simulink model "example_husky"  (R2024b)
settings: Solver=VariableStepAuto  StartTime=0.0  StopTime=inf  RelTol=1e-3
undefined symbols (not defined in the file): gray
settings Model: Creator=tsamak  LastModifiedBy=tsamak
settings OptimizationCC: ZeroExternalMemoryAtStartup=off  ZeroInternalMemoryAtStartup=off  InitFltsAndDblsToZero=on
settings DebuggingCC: UnderSpecifiedDimensionMsg=warning
settings HardwareCC: ProdLongLongMode=on  TargetLongLongMode=on
settings SFSimCC: SimTargetLang=C++  GPUAcceleration=on  SimDLTargetLibrary=cudnn
settings RTWCC: TargetLang=C++  GenerateGPUCode=CUDA  GPUComputeCapability=3.5
settings GRTTargetCC: TargetLangStandard=C++11 (ISO)  CodeInterfacePackaging=C++ class

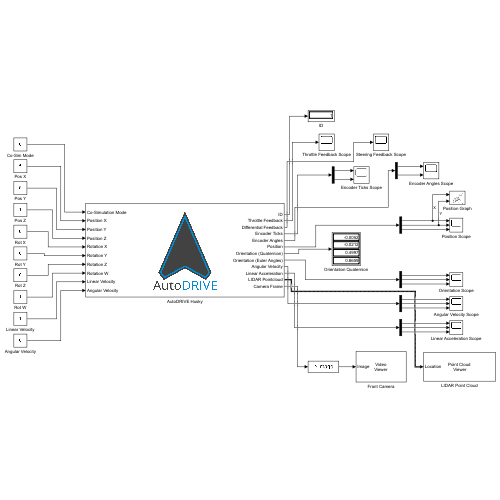
[thumbnail: Simulink's stored preview of the top-level diagram]
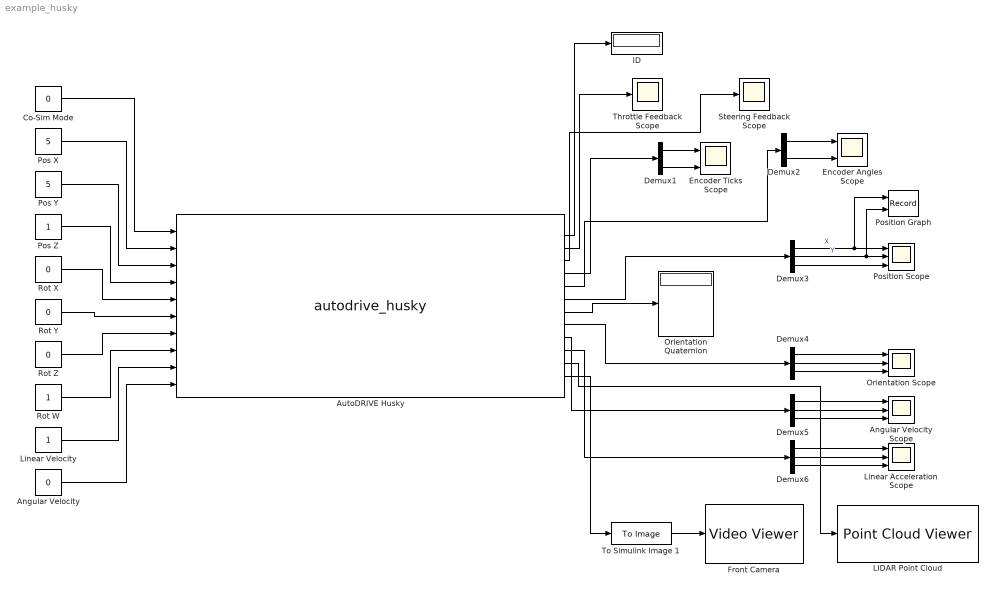
== system example_husky ==
  Angular Velocity : Constant  Value=0
  Angular Velocity Scope : Scope  NumInputPorts=3
  AutoDRIVE Husky : M-S-Function  FunctionName=autodrive_husky  Parameters=Port  mask{Port=4567}
      mask Display:
      | image('autodrive_logo.png');
      | port_label('input', 1, 'Co-Simulation Mode');
      | port_label('input', 2, 'Position X');
      | port_label('input', 3, 'Position Y');
      | port_label('input', 4, 'Position Z');
      | port_label('input', 5, 'Rotation X');
      | port_label('input', 6, 'Rotation Y');
      | port_label('input', 7, 'Rotation Z');
      | port_label('input', 8, 'Rotation W');
      | port_label('input', 9, 'Linear Velocity');
      | port_label('input', 10, 'Angular Velocity');
      | port_label('output', 1, 'ID');
      | port_label('output', 2, 'Throttle Feedback');
      | port_label('output', 3, 'Differential Feedback');
      | port_label('output', 4, 'Encoder Ticks');
      | port_label('output', 5, 'Encoder Angles');
      | port_label('output', 6, 'Position');
      | port_label('output', 7, 'Orientation (Quaternion)');
      | port_label('output', 8, 'Orientation (Euler Angles)');
      | port_label('output', 9, 'Angular Velocity');
      | port_label('output', 10, 'Linear Acceleration');
      | port_label('output', 11, 'LIDAR Pointcloud');
      | port_label('output', 12, 'Camera Frame');
  Co-Sim Mode : Constant  Value=0  OutDataTypeStr=uint8
  Demux1 : Demux  Outputs=2
  Demux2 : Demux  Outputs=2
  Demux{3..6} (4 alike) : Demux  Outputs=3
  Encoder Angles Scope : Scope  NumInputPorts=2
  Encoder Ticks Scope : Scope  NumInputPorts=2
  Front Camera : VideoViewer  colormapValue=gray(256)  FigPos=[11 410 408 304]
  ID : Display
  LIDAR Point Cloud : PointCloudViewer  FigPos=[843.666666666667 412 469.333333333333 328.666666666667]
  Linear Acceleration Scope : Scope  NumInputPorts=3
  Linear Velocity : Constant
  Orientation Quaternion : Display
  Orientation Scope : Scope  NumInputPorts=3
  Pos X : Constant  Value=5
  Pos Y : Constant  Value=5
  Pos Z : Constant
  Position Graph : Record  FileSettingsInternal="{\"entries\":[{\"content\":{\"excelSettings\":{\"content\":{},\"type\":\"Streamout.ExcelSettings\"}},\"type\":\"Streamout.FileSettingStorage\",\"uuid\":\"\"}],\"packageUris\":[\"http:\\/\\/schema.mathworks.com\\/mf0\\/streamout_blocks\\/R2020a\"],\"version\":\"1.0\"}"  Layout=[1 1]  SignalsInternal="{\"entries\":[{\"content\":{\"signals\":[{\"content\":{\"blockPath\":[],\"dimensions\":[1,1],\"domain\":\"\",\"lineColor\":\"#139fff\",\"plots\":[ 1 ],\"port\":1,\"sid\":[\"\"],\"signalID\":1,\"signalName\":\"X\"},\"type\":\"RecordBlkView.Signal\",\"uuid\":\"\"},{\"content\":{\"blockPath\":[],\"dimensions\":[1,1],\"domain\":\"\",\"lineColor\":\"#139fff\",\"plots\":[ 1 ],\"port\":2,\"sid\":[\"\"],\"signalID\":2,\"signalName\":\"Y\"},\"type\":\"RecordBlkView.Signal\",\"uuid\":\"\"}]},\"type\":\"RecordBlkView.InputSignals\",\"uuid\":\"\"}],\"packageUris\":[\"http:\\/\\/schema.mathworks.com\\/mf0\\/streamout_blocks\\/R2020a\"],\"version\":\"1.0\"}"  VisualizationBindings="{\"xyplotplugin\":{\"info\":[{\"series\":[{\"bindingParametersList\":[{\"parameter\":\"X-Axis\",\"signalID\":1,\"signalName\":\"X\"},{\"parameter\":\"Y-Axis\",\"signalID\":2,\"signalName\":\"Y\"}],\"seriesID\":0}],\"subplotID\":1}]}}"  CompatibilityTag=XY
  Position Scope : Scope  NumInputPorts=3
  Rot W : Constant
  Rot X : Constant  Value=0
  Rot Y : Constant  Value=0
  Rot Z : Constant  Value=0
  Steering Feedback Scope : Scope
  Throttle Feedback Scope : Scope
  To Simulink Image 1 : ToImage
  wires:
  Linear Velocity/1 -> AutoDRIVE Husky/9
  Angular Velocity/1 -> AutoDRIVE Husky/10
  Demux3/2 -> Position Scope/2, Position Graph/2  "Y"
  Demux3/1 -> Position Scope/1, Position Graph/1  "X"
  Demux3/3 -> Position Scope/3
  AutoDRIVE Husky/12 -> To Simulink Image 1/1
  To Simulink Image 1/1 -> Front Camera/1
  AutoDRIVE Husky/6 -> Demux3/1
  AutoDRIVE Husky/11 -> LIDAR Point Cloud/1
  AutoDRIVE Husky/1 -> ID/1
  AutoDRIVE Husky/2 -> Throttle Feedback Scope/1
  AutoDRIVE Husky/3 -> Steering Feedback Scope/1
  AutoDRIVE Husky/4 -> Demux1/1
  Demux1/1 -> Encoder Ticks Scope/1
  Demux1/2 -> Encoder Ticks Scope/2
  Demux2/1 -> Encoder Angles Scope/1
  Demux2/2 -> Encoder Angles Scope/2
  AutoDRIVE Husky/5 -> Demux2/1
  Demux4/3 -> Orientation Scope/3
  Demux5/3 -> Angular Velocity Scope/3
  Demux6/3 -> Linear Acceleration Scope/3
  AutoDRIVE Husky/7 -> Orientation Quaternion/1
  AutoDRIVE Husky/8 -> Demux4/1
  AutoDRIVE Husky/9 -> Demux5/1
  AutoDRIVE Husky/10 -> Demux6/1
  Demux4/1 -> Orientation Scope/1
  Demux4/2 -> Orientation Scope/2
  Demux5/1 -> Angular Velocity Scope/1
  Demux5/2 -> Angular Velocity Scope/2
  Demux6/1 -> Linear Acceleration Scope/1
  Demux6/2 -> Linear Acceleration Scope/2
  Rot W/1 -> AutoDRIVE Husky/8
  Rot Z/1 -> AutoDRIVE Husky/7
  Rot Y/1 -> AutoDRIVE Husky/6
  Rot X/1 -> AutoDRIVE Husky/5
  Pos Z/1 -> AutoDRIVE Husky/4
  Pos Y/1 -> AutoDRIVE Husky/3
  Pos X/1 -> AutoDRIVE Husky/2
  Co-Sim Mode/1 -> AutoDRIVE Husky/1
